simulink model "UAV_sync_known_sim"  (R2018b)
settings: Solver=ode23tb  StartTime=0.0  StopTime=35
values from neighbouring files (symbols this model uses):
  C_rho = 1.225    [SC42120_UAV_Preconditions.m]
  D0 = [M0 0 0 0 0 0 ... (first row only)    [SC42120_UAV_Preconditions.m]
  Derivative_gain_phi = 50    [SC42120_UAV_Preconditions.m]
  Derivative_gain_psi = 50    [SC42120_UAV_Preconditions.m]
  Derivative_gain_theta = 50    [SC42120_UAV_Preconditions.m]
  Derivative_gain_x = 50    [SC42120_UAV_Preconditions.m]
  Derivative_gain_y = 50    [SC42120_UAV_Preconditions.m]
  Derivative_gain_z = 50    [SC42120_UAV_Preconditions.m]
  G = 9.80665    [SC42120_UAV_Preconditions.m]
  g0 = [0;0;-M0*G;0;0;0]    [SC42120_UAV_Preconditions.m]
  I0 = [0.02 0 -0.01 ... (first row only)    [SC42120_UAV_Preconditions.m]
  I1 = [0.1 0 -0.01;0 0.05 0;-0.01 0 0.1]    [UAV_sync_known.m]    (also in UAV_sync_unknown.m; UAV_sync_unknown_Node1.m)
  InitWind = [0;0;0]    [SC42120_UAV_Preconditions.m]
  M0 = 10    [SC42120_UAV_Preconditions.m]
  M1 = 20    [UAV_sync_known.m]    (also in UAV_sync_unknown.m; UAV_sync_unknown_Node1.m)
  Proportional_phi = 50    [SC42120_UAV_Preconditions.m]
  Proportional_psi = 50    [SC42120_UAV_Preconditions.m]
  Proportional_theta = 50    [SC42120_UAV_Preconditions.m]
  Proportional_x = 50    [SC42120_UAV_Preconditions.m]
  Proportional_y = 50    [SC42120_UAV_Preconditions.m]
  Proportional_z = 50    [SC42120_UAV_Preconditions.m]
undefined symbols (not defined in the file or in its folder): Aero, APlane, Bxl, C, Ctr, deg, DiscIntNeverNeededParam, F, Guid, Init, Light, MIL, Path, rad, s, Trim, Utility
libraries: aerolibconvert2 x37, simulink x15, dspsigops x7, shared6dof x6, aerolibasang x4, simulink_extras x3, aerolibadyn x1, aerolibtransform2 x1, aerolibwind2 x1
(part 6 of 6)

== matlab function UAV_sync_known_sim/Node 0/VF Approach/PATH FOLLOWING/Straight-line Path Following (Enabled Subsystem)/Vg Estimator/SL_Estimator ==
  data: chi input; chi_d input; chi_q input; e input; param input; Vg input; Vg_hat input; Vg_hat_dot output size=1
function Vg_hat_dot ...
    = estimator (chi, chi_d, chi_q, e, param, Vg, Vg_hat)
%  feedback, der, term2, last_term,diff_chi, diff_2,
%estimator of Vg'
%% Parameters
y_int = param(1);
W = param(2);
Va = param(3);
epsi = param(4);
phiw = param(5);
chi_inf = param(6);
k = param(7);
kk=param(8);
Gamma = param(9);
sigma = param(10);
alpha = param(11);

%% Law

rho = y_int^2/pi^2;   % Positive scale factor used to weight the terms so that y and chi are similar in magnitude

diff_chi = chi-chi_d; % Error of course angle

term =diff_chi/epsi;
if abs(term)<=1
    sat=term;
else
    sat=sign(term);
end

% % derivative of Vg' over x'
der = W*sin(phiw-chi)+(Va^2-W^2*(sin(phiw-chi))^2)^(-0.5)*W^2*sin(phiw-chi)*cos(phiw-chi); % partial derivative of Vg' over chi'

term2 = (-1*chi_inf*2/pi*(k*sin(chi - chi_q))/(1+(k*(e))^2)*Vg_hat);
last_term = -1*kk*sat;

% if Vg_hat - Vg > 1
%     sigma = (Vg_hat - Vg);
% else
%     sigma = 0;
% end

Vg_hat_dot = Gamma/alpha*rho*diff_chi*chi_inf*2/pi*(k*(sin(chi-chi_q)))/(1+(k*(e))^2)...
    - sigma* Gamma * Vg_hat +...
     1*der*(term2/alpha +last_term);



end

== matlab function UAV_sync_known_sim/Node 0/VF Approach/PATH FOLLOWING/Orbit Path Following (Enabled Subsystem)/Compute gamma and distance to center/L.PolarCoord ==
  data: x input; y input; gamma output; c input; d output; chi input
function [gamma, d] = pol_coord(x,y,c,chi)
p = [x,y];
d = sqrt((p(1)-c(1))^2+(p(2)-c(2))^2);
gamma = atan2(p(2)-c(2),p(1)-c(1));

% while gamma - chi < -pi
%     gamma = gamma + 2*pi;
% end
% 
% while gamma - chi > pi
%     gamma = gamma - 2*pi;
% end

end

== matlab function UAV_sync_known_sim/Node 0/VF Approach/PATH MANAGER/Enabled Subsystem/Path Manager ==
  settings: updateMethod=DISCRETE
  data: w input; flag output; x input; y input; origin output; slope output; c output; lambda output; stop_sim output; R input
function [ flag, origin, slope, c, lambda, stop_sim] = fcn( w, x, y, R )
%%
% Index of the current waypoint
persistent i
if isempty(i)
    i = 2;
end
% State = 1 if straight line, state = 2 if orbit
persistent state
if isempty(state)
    state = 1;
end

% Init
n = size(w,1);      % Number of waypoints
flag = 1;           % Switch from SL to orbit
origin = [0 0];
slope = [1 0];
c = [0 0];
lambda = 0;
stop_sim = 0;
z=[0 0];

%%
p = [x y];
q_i_min_1 = (w(i,:)-w(i-1,:)) / norm(w(i,:)-w(i-1,:),2);
q_i = (w(i+1,:)-w(i,:)) / norm(w(i+1,:)-w(i,:),2);
rho = acos(-q_i_min_1*q_i');

if state == 1
    flag = 1;
    origin = w(i-1,:);
    slope = q_i_min_1;
    z = w(i,:) - (R/(tan(rho/2)))*q_i_min_1;
    if (p-z) * q_i_min_1' >= 0
        state = 2;
        %         i=i+1;
    end
    
elseif state == 2
    flag = 0;
    c = w(i,:)-(R/(sin(rho/2)))*(q_i_min_1 - q_i)/(norm(q_i_min_1- q_i));
    %     rho = R;
    lambda = sign(q_i_min_1(1) * q_i(2) - q_i_min_1(2)*q_i(1));
    z = w(i,:) + (R/(tan(rho/2)))*q_i;
    if (p-z) * q_i' >= 0
        i = i + 1;
        state = 1;
    end
end
if i == n-1
    stop_sim = 1;
end

end

== matlab function UAV_sync_known_sim/Node 0/VF Approach/PATH FOLLOWING/Orbit Path Following (Enabled Subsystem)/Loiter Controller/Loiter Controller ==
  data: chi input; y output; chi_d input; d input; Vg input; gamma input; param input
function y  = OrbitController(chi, chi_d, d, Vg, gamma, param)

%%
k = param(1);
kk = param(2);
epsi = param(3);
r = param(4);
j = param(5);
alpha = param(6);

%%
chi_tilde = chi-chi_d;
lt = chi_tilde/epsi;

if abs(lt) <=1
    term = lt;
else
    term = sign(lt);
end

d_tilde = d-r;
beta = k/(1+(k*d_tilde)^2);

err = (chi-gamma);

term2 = Vg /(alpha*d)*sin(err) + j*beta/alpha*Vg*cos(err);

term3 = -kk/alpha*term;

y = chi + term2 + term3;

== matlab function UAV_sync_known_sim/Node 0/VF Approach/PATH FOLLOWING/Orbit Path Following (Enabled Subsystem)/Vg Estimator/Estimator  ==
  data: chi input; d input; gamma input; chi_d input; param input; Vg input; Vg2_hat_dot output size=1; Vg_hat input
function Vg2_hat_dot  = estimator(chi,d,gamma,chi_d, param, Vg, Vg_hat)

%% Parameters
W = param(1);
phiw = param(2);
Va  = param(3);
k  = param(4);
kk = param(5);
epsi = param(6);
d_int = param(7);
R  = param(8);
j = param(9);
Gamma = param(10);
sigma = param(11);

%% Estimator of Vg'

err_1 = (phiw - chi);
err_2 = chi - gamma;
chi_tilde = chi - chi_d;

term = chi_tilde / epsi;
rho = (d_int / pi)^2;

if abs(term) <= 1
    chi_tilde_eps = term;
else
    chi_tilde_eps = sign(term);
end

if Vg_hat - Vg > 0.5 ||  Vg_hat - Vg < -0.5
    sigma = 3*(Vg_hat - Vg);
else
    sigma = 0;
end


% Partial derivative of Vg' over chi'
beta = k/(1 + (k * (d - R))^2);
der = W * sin(err_1) + (Va^2 - W^2 * (sin(err_1))^2)^(-0.5) * W^2 * sin(err_1) * cos(err_1); 

term1 = -Gamma * rho * (chi_tilde) * (sin(err_2) / d + j * beta * cos(err_2));
term2 = der*(Vg_hat*sin(err_2)/d + j*beta*Vg_hat*cos(err_2) - kk*chi_tilde_eps);
Vg2_hat_dot =  term1 + 1*term2 - sigma*Gamma*Vg_hat;
end
